simulink model "Sist_stab_H_vozm"  (R2018b)
settings: Solver=VariableStepAuto  StartTime=0.0  StopTime=10.0  RelTol=1e-3
libraries: simulink x2
settings Model: Creator=Танечка  LastModifiedBy=Танечка

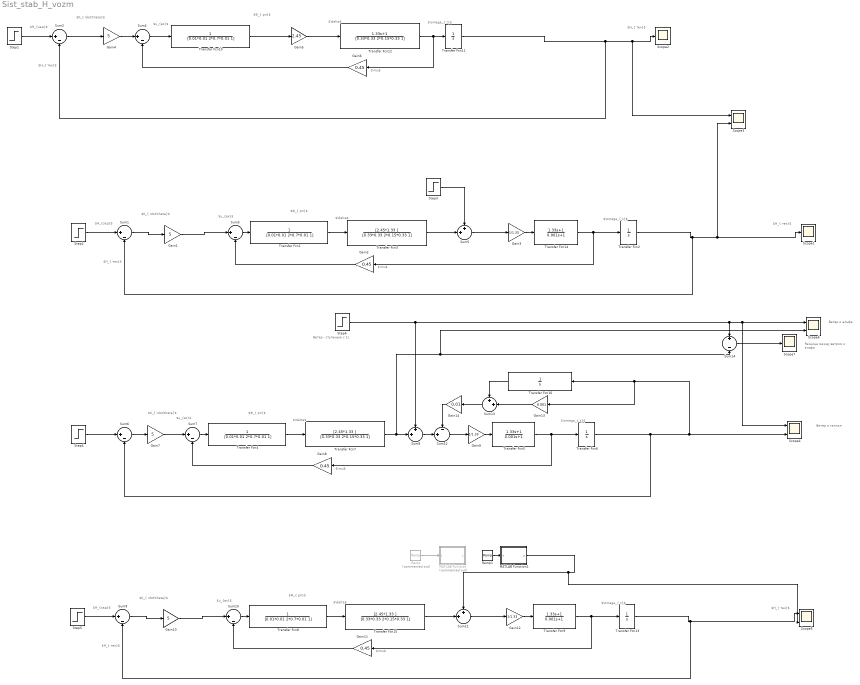
== system Sist_stab_H_vozm ==
  note: Ветер - ступенька с 1с
  note: $\delta$
  note: $K_{ \dot\theta}$
  note: $u_{вх}$
  note: $H_{ тек}$
  note: $\mu$
  note: $Ф_{ рп}$
  note: $\omega_{ z}$
  note: $H_{зад}$
  note: $H_{ тек}$
  note: $\omega_{ z}$
  note: $H_{ тек}$
  note: $H_{ тек}$
  note: $Ф_{ рп}$
  note: $u_{вх}$
  note: $K_{ \dot\theta}$
  note: $\mu$
  note: $\delta$
  note: $H_{зад}$
  note: $Ф_{ рп}$
  note: $u_{вх}$
  note: $\mu$
  note: $\delta$
  note: $K_{ \dot\theta}$
  note: $\omega_{ z}$
  note: $H_{ тек}$
  note: $u_{вх}$
  note: $\delta$
  note: $K_{ \dot\theta}$
  note: $H_{ тек}$
  note: $Ф_{ рп}$
  note: $\mu$
  note: $\omega_{ z}$
  note: $H_{зад}$
  note: Разница между
      | ветром и альфа
  note: Ветер и
      | альфа
  note: Ветер и
      | тангаж
  Gain{1,4,7,10} (4 alike) : Gain  Gain=5
  Gain{2,6,8,11} (4 alike) : Gain  Gain=0.45
  Gain12 : Gain  Gain=1/1.33
  Gain13 : Gain  Gain=0.001
  Gain14 : Gain  Gain=0.01
  Gain3 : Gain  Gain=1/1.33
  Gain5 : Gain  Gain=2.45
  Gain9 : Gain  Gain=1/1.33
  MATLAB Function : MATLAB Function  Commented=on  TreatAsAtomicUnit=on
  MATLAB Function1 : MATLAB Function  TreatAsAtomicUnit=on
  Ramp : simulink/Sources/Ramp  Commented=on  slope=1  start=0  InitialOutput=0
  Ramp1 : simulink/Sources/Ramp  slope=1  start=0  InitialOutput=0
  Scope1 : Scope
  Scope2 : Scope
  Scope{3..6} (4 alike) : Scope  NumInputPorts=2
  Scope7 : Scope
  Step1 : Step  SampleTime=0
  Step2 : Step  Time=0  SampleTime=0
  Step3 : Step  After=3  SampleTime=0
  Step4 : Step  Time=0  After=0  SampleTime=0
  Step5 : Step  Time=0  SampleTime=0
  Step6 : Step  After=3  SampleTime=0
  Sum{1..4,6..7,9..10} (8 alike) : Sum  Inputs=|+-
  Sum{5,8,11,13} (4 alike) : Sum  Inputs=++|
  Sum12 : Sum  Inputs=-+|
  Sum14 : Sum  Inputs=+|-
  Transfer Fcn{1,4,8,10} (4 alike) : TransferFcn  Numerator=[ 1]  Denominator=[0.01*0.01 2*0.7*0.01 1]
  Transfer Fcn{2,6,11,13,16} (5 alike) : TransferFcn  Denominator=[1 0]
  Transfer Fcn12 : TransferFcn  Numerator=[1.33 1]  Denominator=[0.33*0.33 2*0.15*0.33 1]
  Transfer Fcn14 : TransferFcn  Numerator=[1.33 1 ]  Denominator=[0.001 1]
  Transfer Fcn15 : TransferFcn  Numerator=[2.45*1.33 ]  Denominator=[0.33*0.33 2*0.15*0.33 1]
  Transfer Fcn3 : TransferFcn  Numerator=[2.45*1.33 ]  Denominator=[0.33*0.33 2*0.15*0.33 1]
  Transfer Fcn5 : TransferFcn  Numerator=[1.33 1 ]  Denominator=[0.001 1]
  Transfer Fcn7 : TransferFcn  Numerator=[2.45*1.33 ]  Denominator=[0.33*0.33 2*0.15*0.33 1]
  Transfer Fcn9 : TransferFcn  Numerator=[1.33 1 ]  Denominator=[0.001 1]
  wires:
  Step1/1 -> Sum2/1
  Transfer Fcn11/1 -> Sum2/2, Scope3/1, Scope2/1
  Sum2/1 -> Gain4/1
  Transfer Fcn10/1 -> Gain5/1
  Gain4/1 -> Sum4/1
  Gain6/1 -> Sum4/2
  Transfer Fcn12/1 -> Gain6/1, Transfer Fcn11/1
  Sum1/1 -> Gain1/1
  Gain2/1 -> Sum3/2
  Gain1/1 -> Sum3/1
  Transfer Fcn1/1 -> Transfer Fcn3/1
  Transfer Fcn2/1 -> Scope3/2, Scope1/1, Sum1/2
  Sum3/1 -> Transfer Fcn1/1
  Step2/1 -> Sum1/1
  Gain3/1 -> Transfer Fcn14/1
  Transfer Fcn14/1 -> Gain2/1, Transfer Fcn2/1
  Sum4/1 -> Transfer Fcn10/1
  Gain5/1 -> Transfer Fcn12/1
  Transfer Fcn3/1 -> Sum5/2
  Sum5/1 -> Gain3/1
  Step3/1 -> Sum5/1
  Gain7/1 -> Sum7/1
  Gain9/1 -> Transfer Fcn5/1
  Gain8/1 -> Sum7/2
  Transfer Fcn4/1 -> Transfer Fcn7/1
  Sum6/1 -> Gain7/1
  Transfer Fcn5/1 -> Gain8/1, Transfer Fcn6/1
  Sum7/1 -> Transfer Fcn4/1
  Step4/1 -> Sum6/1
  Transfer Fcn6/1 -> Sum6/2, Transfer Fcn16/1, Gain13/1, Scope4/2
  Ramp/1 -> MATLAB Function/1(t)
  Ramp1/1 -> MATLAB Function1/1(t)
  MATLAB Function1/1(y) -> Scope5/2, Sum11/1
  Step5/1 -> Sum9/1
  Transfer Fcn15/1 -> Sum11/2
  Sum10/1 -> Transfer Fcn8/1
  Gain12/1 -> Transfer Fcn9/1
  Transfer Fcn13/1 -> Scope5/1, Sum9/2
  Transfer Fcn9/1 -> Gain11/1, Transfer Fcn13/1
  Sum9/1 -> Gain10/1
  Gain11/1 -> Sum10/2
  Gain10/1 -> Sum10/1
  Transfer Fcn8/1 -> Transfer Fcn15/1
  Sum11/1 -> Gain12/1
  Gain13/1 -> Sum13/2
  Transfer Fcn16/1 -> Sum13/1
  Sum13/1 -> Gain14/1
  Step6/1 -> Sum14/1, Scope4/1, Scope6/1, Sum8/1
  Transfer Fcn7/1 -> Sum8/2, Sum14/2, Scope6/2
  Sum14/1 -> Scope7/1
  Sum8/1 -> Sum12/2
  Sum12/1 -> Gain9/1
  Gain14/1 -> Sum12/1

== matlab function Sist_stab_H_vozm/MATLAB Function1 ==
  data: t input; y output
function y = fcn(t)

%     if t>= 1 && t<=2
% 
%         y = 3;
%     else
%         y = 0;
%     end

    if t>= 1

        y = 3;
    else
        y = 3*t;
    end
    
    
    

end

== matlab function Sist_stab_H_vozm/MATLAB Function ==
  data: t input; y output
function y = fcn(t)

    if t>= 1 && t<=2

        y = 3;
    else
        y = 0;
    end
    
    

end
